simulink model "TestEnvironment"  (R2015b)
settings: Solver=VariableStepAuto  StartTime=0.0  StopTime=200.0  RelTol=1e-3
libraries: simulink x2
settings Model: Creator=ndoehlert  LastModifiedBy=dominic

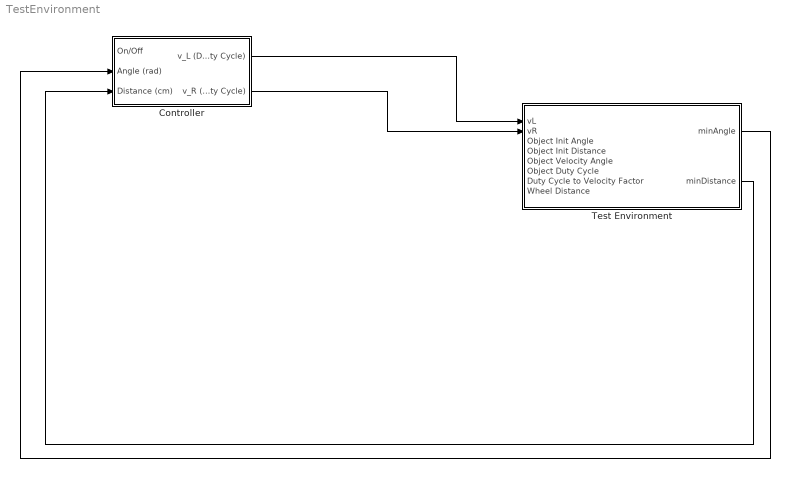
== system TestEnvironment ==
  Controller : Subsystem
  Test Environment : Subsystem
  wires:
  Controller/1(v_L (Duty Cycle)) -> Test Environment/1(vL)
  Controller/2(v_R (Duty Cycle)) -> Test Environment/2(vR)
  Test Environment/2(minDistance) -> Controller/3(Distance (cm))
  Test Environment/1(minAngle) -> Controller/2(Angle (rad))

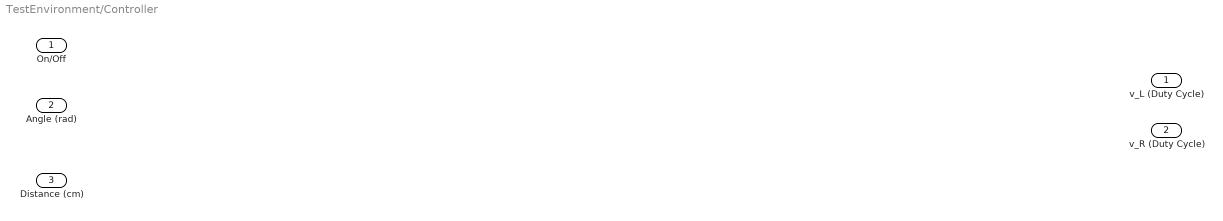
== system TestEnvironment/Controller ==
  On/Off : Inport
  Angle (rad) : Inport  Port=2
  Distance (cm) : Inport  Port=3
  v_L (Duty Cycle) : Outport
  v_R (Duty Cycle) : Outport  Port=2

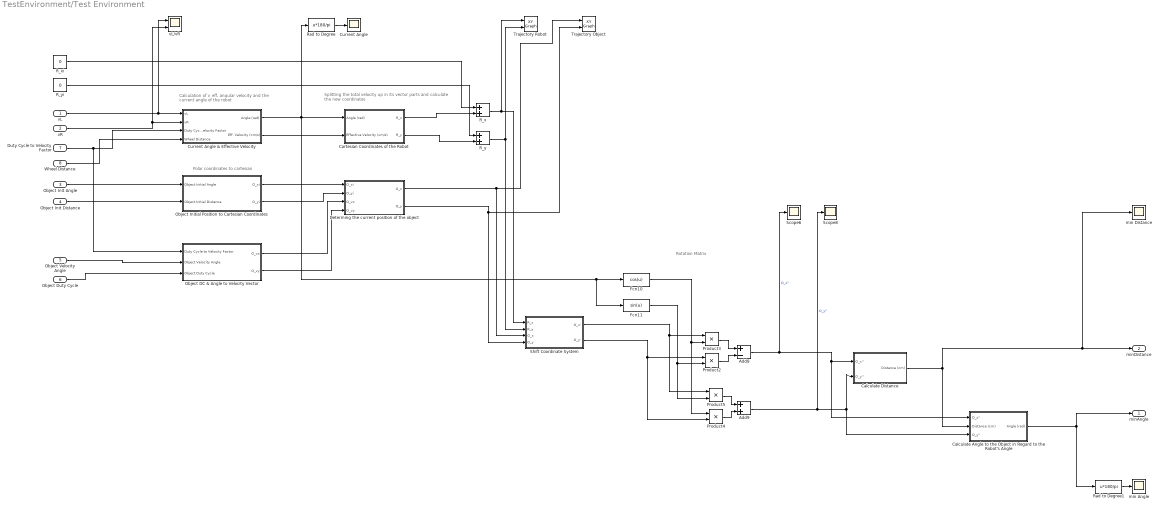
== system TestEnvironment/Test Environment ==
  note: Splitting the total velocity up in its vector parts and calculate
      | the new coordinates
  note: Calculation of v_eff, angular velocity and the
      | current angle of the robot
  note: Rotation Matrix
  note: Polar coordinates to cartesian
  vL : Inport
  vR : Inport  Port=2
  Object Init Angle : Inport  Port=3
  Object Init Distance : Inport  Port=4
  Object Velocity Angle : Inport  Port=5
  Object Duty Cycle : Inport  Port=6
  Duty Cycle to Velocity Factor : Inport  Port=7
  Wheel Distance : Inport  Port=8
  Add8 : Sum  Inputs=+-
  Add9 : Sum
  Calculate Angle to the Object in Regard to the Robot's Angle : Subsystem
  Calculate Distance : Subsystem
  Cartesian Coordinates of the Robot : Subsystem
  Current Angle : Scope
  Current Angle & Effective Velocity : Subsystem
  Determing the current position of the object : Subsystem
  Fcn10 : Fcn  Expr=cos(u)
  Fcn11 : Fcn  Expr=sin(u)
  Object DC & Angle to Velocity Vector : Subsystem
  Object Initial Position to Cartesian Coordinates : Subsystem
  Product{2..5} (4 alike) : Product
  R_x : Sum
  R_xi : Constant  Value=0
  R_y : Sum
  R_yi : Constant  Value=0
  Rad to Degree : Fcn  Expr=u*180/pi
  Rad to Degree1 : Fcn  Expr=u*180/pi
  Scope6 : Scope
  Scope8 : Scope
  Shift Coordinate System : Subsystem
  Trajectory Object : simulink/Sinks/XY Graph  xmin=-500  xmax=500  ymin=-500  ymax=500  st=-1
  Trajectory Robot : simulink/Sinks/XY Graph  xmin=-500  xmax=500  ymin=-500  ymax=500  st=-1
  min Angle : Scope
  min Distance : Scope
  vL/vR : Scope  NumInputPorts=2
  minAngle : Outport
  minDistance : Outport  Port=2
  wires:
  vL/1 -> vL/vR/1, Current Angle & Effective Velocity/1(vL)
  vR/1 -> Current Angle & Effective Velocity/2(vR), vL/vR/2
  R_xi/1 -> R_x/1
  R_yi/1 -> R_y/1
  R_x/1 -> Shift Coordinate System/1(R_x), Trajectory Robot/1
  R_y/1 -> Shift Coordinate System/2(R_y), Trajectory Robot/2
  Duty Cycle to Velocity Factor/1 -> Current Angle & Effective Velocity/3(Duty Cycle to Velocity Factor), Object DC & Angle to Velocity Vector/1(Duty Cycle to Velocity Factor)
  Rad to Degree/1 -> Current Angle/1
  Fcn10/1 -> Product4/1, Product3/2
  Fcn11/1 -> Product5/2, Product2/2
  Product3/1 -> Add8/1
  Product2/1 -> Add8/2
  Product5/1 -> Add9/1
  Product4/1 -> Add9/2
  Add8/1 -> Calculate Angle to the Object in Regard to the Robot's Angle/1(O_x''), Calculate Distance/1(O_x''), Scope6/1  "O_x''"
  Add9/1 -> Calculate Angle to the Object in Regard to the Robot's Angle/3(O_y''), Calculate Distance/2(O_y''), Scope8/1  "O_y''"
  Rad to Degree1/1 -> min Angle/1
  Current Angle & Effective Velocity/1(Angle (rad)) -> Fcn11/1, Fcn10/1, Cartesian Coordinates of the Robot/1(Angle (rad)), Rad to Degree/1
  Wheel Distance/1 -> Current Angle & Effective Velocity/4(Wheel Distance)
  Current Angle & Effective Velocity/2(Eff. Velocity (cm/s)) -> Cartesian Coordinates of the Robot/2(Effective Velocity (cm/s))
  Cartesian Coordinates of the Robot/1(R_x) -> R_x/2
  Cartesian Coordinates of the Robot/2(R_y) -> R_y/2
  Object Init Angle/1 -> Object Initial Position to Cartesian Coordinates/1(Object Initial Angle)
  Object Init Distance/1 -> Object Initial Position to Cartesian Coordinates/2(Object Initial Distance)
  Object Velocity Angle/1 -> Object DC & Angle to Velocity Vector/2(Object Velocity Angle)
  Object Duty Cycle/1 -> Object DC & Angle to Velocity Vector/3(Object Duty Cycle)
  Determing the current position of the object/2(O_y) -> Shift Coordinate System/4(O_y), Trajectory Object/2
  Determing the current position of the object/1(O_x) -> Shift Coordinate System/3(O_x), Trajectory Object/1
  Object Initial Position to Cartesian Coordinates/1(O_xi) -> Determing the current position of the object/1(O_xi)
  Object Initial Position to Cartesian Coordinates/2(O_yi) -> Determing the current position of the object/2(O_yi)
  Object DC & Angle to Velocity Vector/1(O_vx) -> Determing the current position of the object/3(O_vx)
  Object DC & Angle to Velocity Vector/2(O_vy) -> Determing the current position of the object/4(O_vy)
  Shift Coordinate System/2(O_y') -> Product4/2, Product2/1
  Shift Coordinate System/1(O_x') -> Product5/1, Product3/1
  Calculate Distance/1(Distance (cm)) -> Calculate Angle to the Object in Regard to the Robot's Angle/2(Distance (cm)), min Distance/1, minDistance/1
  Calculate Angle to the Object in Regard to the Robot's Angle/1(Angle (rad)) -> minAngle/1, Rad to Degree1/1

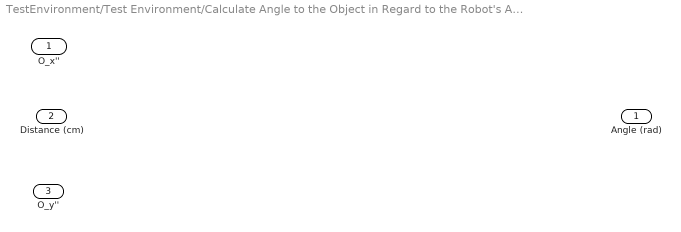
== system TestEnvironment/Test Environment/Calculate Angle to the Object in Regard to the Robot's Angle ==
  O_x'' : Inport
  Distance (cm) : Inport  Port=2
  O_y'' : Inport  Port=3
  Angle (rad) : Outport

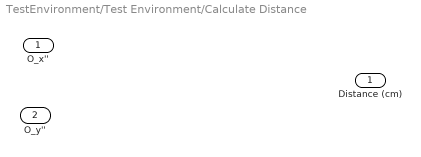
== system TestEnvironment/Test Environment/Calculate Distance ==
  O_x'' : Inport
  O_y'' : Inport  Port=2
  Distance (cm) : Outport

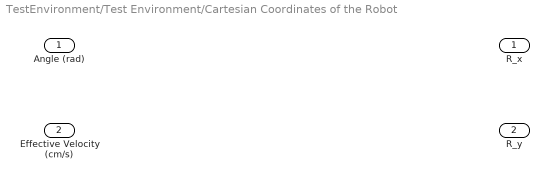
== system TestEnvironment/Test Environment/Cartesian Coordinates of the Robot ==
  Angle (rad) : Inport
  Effective Velocity (cm/s) : Inport  Port=2
  R_x : Outport
  R_y : Outport  Port=2

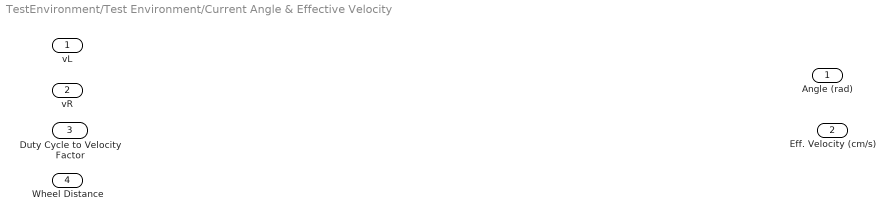
== system TestEnvironment/Test Environment/Current Angle & Effective Velocity ==
  vL : Inport
  vR : Inport  Port=2
  Duty Cycle to Velocity Factor : Inport  Port=3
  Wheel Distance : Inport  Port=4
  Angle (rad) : Outport
  Eff. Velocity (cm/s) : Outport  Port=2

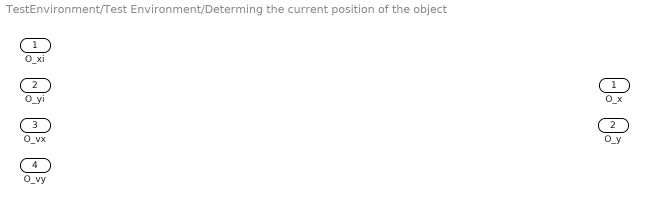
== system TestEnvironment/Test Environment/Determing the current position of the object ==
  O_xi : Inport
  O_yi : Inport  Port=2
  O_vx : Inport  Port=3
  O_vy : Inport  Port=4
  O_x : Outport
  O_y : Outport  Port=2

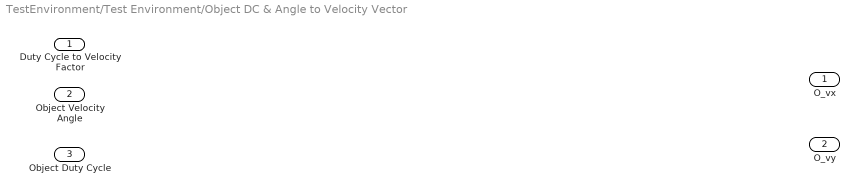
== system TestEnvironment/Test Environment/Object DC & Angle to Velocity Vector ==
  Duty Cycle to Velocity Factor : Inport
  Object Velocity Angle : Inport  Port=2
  Object Duty Cycle : Inport  Port=3
  O_vx : Outport
  O_vy : Outport  Port=2

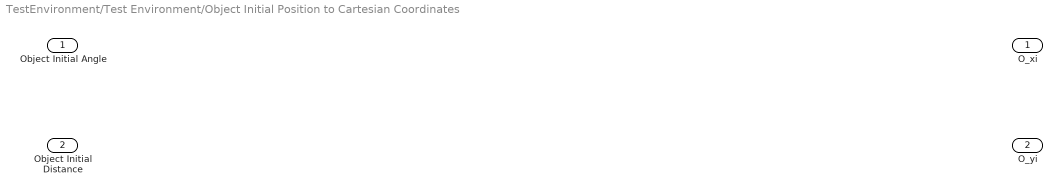
== system TestEnvironment/Test Environment/Object Initial Position to Cartesian Coordinates ==
  Object Initial Angle : Inport
  Object Initial Distance : Inport  Port=2
  O_xi : Outport
  O_yi : Outport  Port=2

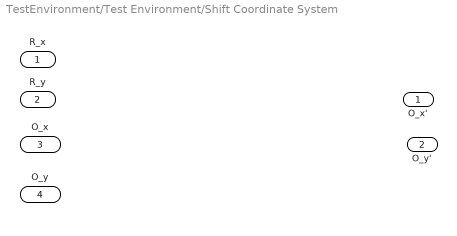
== system TestEnvironment/Test Environment/Shift Coordinate System ==
  R_x : Inport
  R_y : Inport  Port=2
  O_x : Inport  Port=3
  O_y : Inport  Port=4
  O_x' : Outport
  O_y' : Outport  Port=2
